simulink subsystem "integrator_sl"  (R2026a)
settings: Solver=VariableStepAuto
model mask{Mass=0, Inertia=0, Pos=0, Velocity=0, Orient=0, AngVelocity=0}
  mask prompts: Mass "Mass [kg]"; Inertia "Inertia matrix (3x3)"; Pos "Initial Position (NED)"; Velocity "Initial velocity (BODY)"; Orient "Initial Orientation (NED)"; AngVelocity "Angular velocity (BODY)"
libraries: aerolibutil x2, matrix_library x2, sharedutil x1
settings Model: Creator=User  LastModifiedBy=User

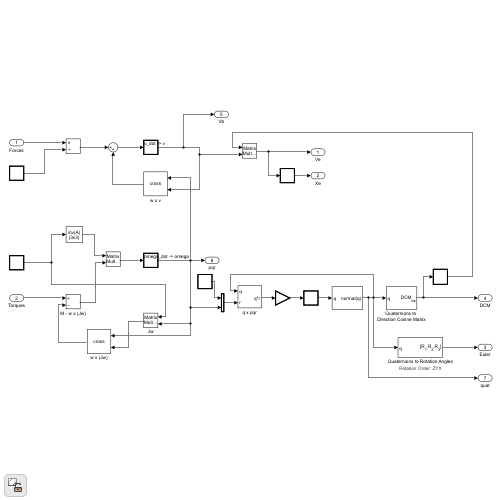
[thumbnail: Simulink's stored preview of the top-level diagram]
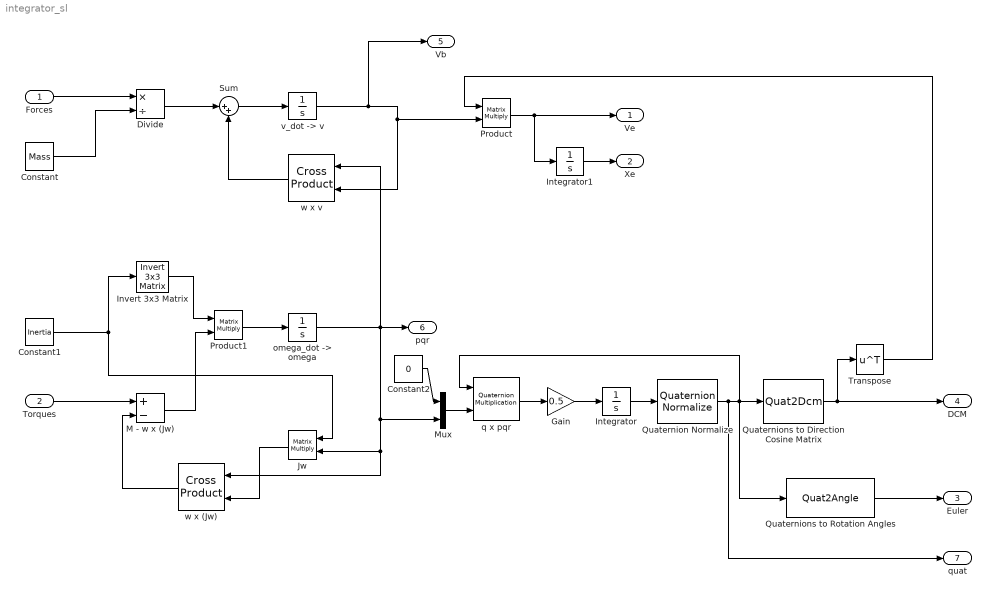
== system integrator_sl ==
  Forces : Inport
  Torques : Inport  Port=2
  Constant : Constant  Value=Mass
  Constant1 : Constant  Value=Inertia
  Constant2 : Constant  Value=0
  Divide : Product  Inputs=*/
  Gain : Gain  Gain=0.5
  Integrator : Integrator  InitialCondition="eul2quat(Orient, \"ZYX\");"
  Integrator1 : Integrator  InitialCondition=Pos
  Invert 3x3 Matrix : aerolibutil/Invert  3x3 Matrix
  Jw : Product  Multiplication=Matrix(*)
  M - w x (Jw) : Sum  Inputs=+-
  Mux : Mux  Inputs=2
  Product : Product  Multiplication=Matrix(*)
  Product1 : Product  Multiplication=Matrix(*)
  Quaternion Normalize : sharedutil/Quaternion Normalize  aMode=aMode
  Quaternions to Direction Cosine Matrix : Quat2Dcm
  Quaternions to Rotation Angles : Quat2Angle
      settings: AttributesFormatString=Rotation Order: %<rotationOrder>
  Sum : Sum  Inputs=|++
  Transpose : Math  Operator=transpose
  "omega_dot -> omega" : Integrator  InitialCondition=AngVelocity
  q x pqr : aerolibutil/Quaternion Multiplication
  "v_dot -> v" : Integrator  InitialCondition=Velocity
  w x (Jw) : matrix_library/Cross Product
  w x v : matrix_library/Cross Product
  Ve : Outport
  Xe : Outport  Port=2
  Euler : Outport  Port=3
  DCM : Outport  Port=4
  Vb : Outport  Port=5
  pqr : Outport  Port=6
  quat : Outport  Port=7
  wires:
  Constant/1 -> Divide/2
  Forces/1 -> Divide/1
  Divide/1 -> Sum/1
  w x v/1 -> Sum/2
  Sum/1 -> "v_dot -> v"/1
  "v_dot -> v"/1 -> Vb/1, w x v/2, Product/2
  Constant1/1 -> Jw/1, Invert 3x3 Matrix/1
  "omega_dot -> omega"/1 -> w x v/1, pqr/1, Mux/2, w x (Jw)/1, Jw/2
  Torques/1 -> M - w x (Jw)/1
  Jw/1 -> w x (Jw)/2
  w x (Jw)/1 -> M - w x (Jw)/2
  Invert 3x3 Matrix/1 -> Product1/1
  M - w x (Jw)/1 -> Product1/2
  Product1/1 -> "omega_dot -> omega"/1
  q x pqr/1 -> Gain/1
  Gain/1 -> Integrator/1
  Product/1 -> Integrator1/1, Ve/1
  Integrator1/1 -> Xe/1
  Quaternions to Rotation Angles/1 -> Euler/1
  Constant2/1 -> Mux/1
  Transpose/1 -> Product/1
  Integrator/1 -> Quaternion Normalize/1
  Quaternions to Direction Cosine Matrix/1 -> Transpose/1, DCM/1
  Quaternion Normalize/1 -> Quaternions to Rotation Angles/1, Quaternions to Direction Cosine Matrix/1, q x pqr/1, quat/1
  Mux/1 -> q x pqr/2
